simulink model "hw3"  (Simulink 7.9)
settings: Solver=ode45  StartTime=0.0  StopTime=20  RelTol=1e-3
settings Model: Creator=bazkoale  LastModifiedBy=alex
settings DataIOCC: SignalLoggingSaveFormat=Dataset
settings OptimizationCC: ExpressionDepthLimit=128
settings DebuggingCC: MultiTaskDSMMsg=warning  MultiTaskCondExecSysMsg=none  StrictBusMsg=None
settings RTWCC: IncludeERTFirstTime=on
settings CodeAppCC: CustomSymbolStrType=$N$R$M_T

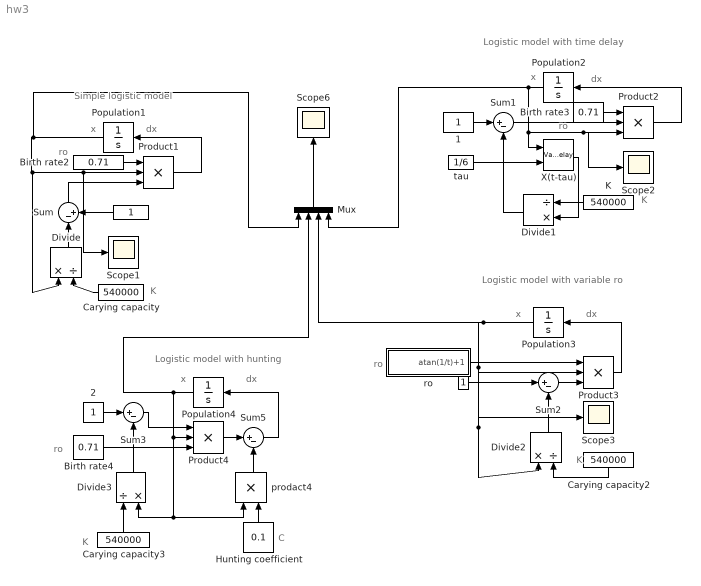
== system hw3 ==
  note: x
  note: dx
  note: dx
  note: x
  note: dx
  note: x
  note: dx
  note: Simple logistic model
  note: Logistic model with hunting
  note: x
  note: Logistic model with time delay
  note: K
  note: Logistic model with variable ro
  note: K
  note: K
  note: ro
  note: ro
  note: ro
  note: ro
  note: K
  note: C
  " " : Constant
  "  " : Constant
  "  2" : Constant
  " 1" : Constant
  " tau" : Constant  Value=1/6
  " Scope6" : Scope
      settings: ShowLegends=on
  Birth rate2 : Constant  Value=0.71
  Birth rate3 : Constant  Value=0.71
  Birth rate4 : Constant  Value=0.71
  Carying capacity : Constant  Value=540000
  Carying capacity2 : Constant  Value=540000
  Carying capacity3 : Constant  Value=540000
  Divide : Product  Inputs=*/
  Divide1 : Product  Inputs=/*
  Divide2 : Product  Inputs=*/
  Divide3 : Product  Inputs=/*
  Hunting coefficient : Constant  Value=0.1
  K : Constant  Value=540000
  Mux : Mux
  Population{1..4} (4 alike) : Integrator  InitialCondition=540000/4
  Product{1..4} (4 alike) : Product  Inputs=3
  Scope1 : Scope
      settings: SaveName=ScopeData3
  Scope2 : Scope
      settings: SaveName=ScopeData2
  Scope3 : Scope
      settings: SaveName=ScopeData6
  Sum : Sum  Inputs=|-+
  Sum{1..3,5} (4 alike) : Sum  Inputs=|+-
  X(t-tau) : VariableTransportDelay  MaximumDelay=10
  "prodact4 " : Product  Inputs=**
  ro : Subsystem
  wires:
  Population1/1 -> Divide/1, Product1/2, Scope1/1, Mux/1
  Product1/1 -> Population1/1
  Divide1/1 -> Sum1/2
  Product2/1 -> Population2/1
  " tau"/1 -> X(t-tau)/2
  Birth rate2/1 -> Product1/1
  Sum/1 -> Product1/3
  Divide2/1 -> Sum2/2
  Product3/1 -> Population3/1
  Sum2/1 -> Product3/3
  ro/1("atan(1/t)+1 ") -> Product3/1
  "  "/1 -> Sum2/1
  "  2"/1 -> Sum3/1
  Divide3/1 -> Sum3/2
  Hunting coefficient/1 -> "prodact4 "/2
  Carying capacity3/1 -> Divide3/1
  Product4/1 -> Sum5/1
  Mux/1 -> " Scope6"/1
  Carying capacity2/1 -> Divide2/2
  Sum3/1 -> Product4/1
  Birth rate4/1 -> Product4/3
  "prodact4 "/1 -> Sum5/2
  Population4/1 -> Product4/2, Divide3/2, "prodact4 "/1, Mux/2
  Sum5/1 -> Population4/1
  K/1 -> Divide1/1
  " 1"/1 -> Sum1/1
  Population2/1 -> X(t-tau)/1, Scope2/1, Product2/3, Mux/4
  Birth rate3/1 -> Product2/1
  Sum1/1 -> Product2/2
  X(t-tau)/1 -> Divide1/2
  Population3/1 -> Product3/2, Divide2/1, Scope3/1, Mux/3
  Carying capacity/1 -> Divide/2
  Divide/1 -> Sum/1
  " "/1 -> Sum/2

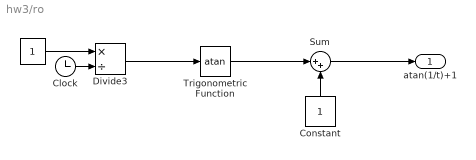
== system hw3/ro ==
  " " : Constant
  Clock : Clock
  Constant : Constant
  Divide3 : Product  Inputs=*/
  Sum : Sum  Inputs=|++
  Trigonometric Function : Trigonometry  Operator=atan
  "atan(1/t)+1 " : Outport
  wires:
  " "/1 -> Divide3/1
  Clock/1 -> Divide3/2
  Divide3/1 -> Trigonometric Function/1
  Trigonometric Function/1 -> Sum/1
  Constant/1 -> Sum/2
  Sum/1 -> "atan(1/t)+1 "/1
